simulink model "DC_Microgrid_Final"  (R2024b)
settings: Solver=VariableStepAuto  StartTime=0.0  StopTime=1.2  RelTol=1e-3
undefined symbols (not defined in the file): Ion, Lithium
libraries: spsSeriesRLCBranchLib x12, spsMeanLib x12, spsCurrentMeasurementLib x9, spsMosfetLib x9, spsIGBTDiodeLib x4, spsStairGeneratorLib x4, spsPWMGeneratorDCDCLib x4, spsVoltageMeasurementLib x3, slpidlib x3, spsDiodeLib x2, spsThreePhaseVIMeasurementLib x1, spsUniversalBridgeLib x1
settings Model: Creator=MCHJOH015  LastModifiedBy=MCHJOH015
settings SolverCC: ZeroCrossAlgorithm=Adaptive
settings DebuggingCC: MaxConsecutiveZCsMsg=none  MaskedZcDiagnostic=none  IgnoredZcDiagnostic=none

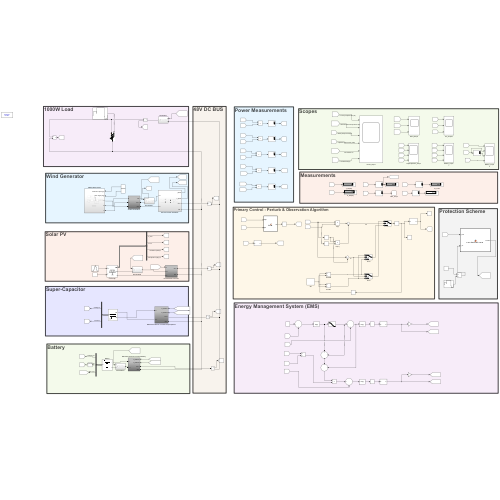
[thumbnail: Simulink's stored preview of the top-level diagram]
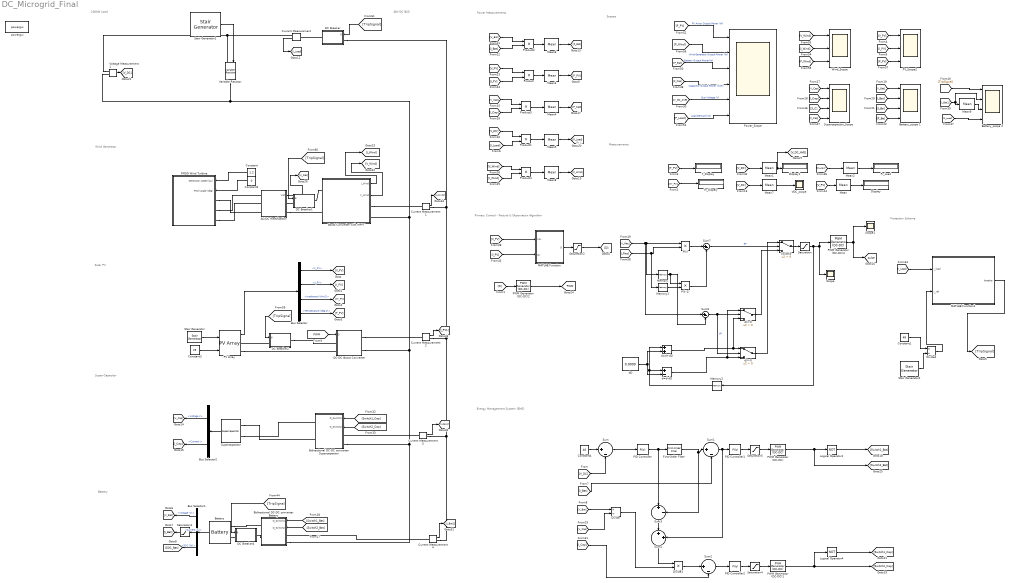
== system DC_Microgrid_Final ==
  note: Pr_L
  note: Power Measurements
  note: Scopes
  note: Protection Scheme
  note: Measurements
  note: Primary Control - Perturb & Observation Algorithm
  note: Super-Capacitor
  note: Solar PV
  note: Wind Generator
  note: 1000W Load
  note: 48V DC BUS
  note: Energy Management System (EMS)
  note: Battery
  AC/DC Rectification : Subsystem
  Battery : spsBatteryLib/Battery  BatType=Lithium-Ion  NomV=25.6  NomQ=200  SOC=50  Batt_Tr=0.1  PresetModel=on  MaxQ=200  MinV=19.2  FullV=29.7981  Dis_rate=86.9565  R=0.00128  Normal_OP=180.8696  expZone="[27.6579      9.82609]"
      settings: LibrarySourceBlock=electricdrivelib/Extra Sources/Battery
  Battery_scope 1 : Scope  NumInputPorts=4
  Battery_scope 2 : Scope  NumInputPorts=4
  Bidirectional DC-DC converter Battery : Subsystem
  Bidirectional DC-DC converter Supercapacitor : Subsystem
  Boost Converter with MPPT : Subsystem
  Bus Selector : BusSelector  OutputSignals=V_PV,I_PV,Irradiance (W/m2),Temperature (deg C)
  Bus Selector1 : BusSelector  OutputSignals=Voltage (V),Current (A),SOC (%)
  Bus Selector2 : BusSelector  OutputSignals=Voltage V,Current I
  Constant : Constant  Value=1.2
  Constant1 : Constant  Value=48
  Constant2 : Constant  Value=0
  Constant3 : Constant  Value=25
  Constant4 : Constant  Value=48
  Current Measurement{,1..4} (5 alike) : spsCurrentMeasurementLib/Current Measurement  PhasorSimulation=off  OutputType=Complex  PSBequivalent=0
  DC Breaker : Subsystem
  DC Breaker1 : Subsystem
  DC Breaker2 : Subsystem
  DC Breaker4 : Subsystem
  DC-DC Boost Converter : Subsystem
  Display : Display
  Display1 : Display
  Divide : Product  Inputs=*/
  Divide1 : Product  Inputs=**
  Divide2 : Product  Inputs=*/
  First-Order Filter : spsFirstOrderFilterLib/First-Order Filter  FilterType=Lowpass  Tc=0.015  Ts=0  Initialize=off  Vac_Init=[0, 0, 60]  Vdc_Init=0  PlotResponse=off  FreqRange="[0,  200,  1]"
  Irr_Dispaly : Display
  Logical Operator1 : Logic  Operator=NOT  IconShape=distinctive  AllPortsSameDT=off  OutDataTypeStr=boolean
  Logical Operator4 : Logic  Operator=NOT  IconShape=distinctive  AllPortsSameDT=off  OutDataTypeStr=boolean
  MATLAB Function : MATLAB Function  TreatAsAtomicUnit=on
  MATLAB Function1 : MATLAB Function  TreatAsAtomicUnit=on
  Mean{,1..9} (10 alike) : spsMeanLib/Mean  Freq=60  Vinit=0  Ts=0
  Memory : Memory  InheritSampleTime=on  LinearizeAsDelay=on
  Memory1 : Memory  InheritSampleTime=on  LinearizeAsDelay=on
  Memory2 : Memory
  P(k) : Product
  P(k-1) : Product
  PID Controller : slpidlib/PID Controller  Controller=PI  Form=Parallel  TimeDomain=Continuous-time  UseExternalTs=off  SampleTime=-1  IntegratorMethod=Forward Euler  FilterMethod=Forward Euler  ControllerParametersSource=internal  P=1.47  I=3088.21  UseKiTs=off  D=0  UseExternalDerivativeSource=off  N=100  UseFilter=on  TunerSelectOption=Transfer Function Based (PID Tuner App)  InitialConditionSource=internal  InitialConditionForIntegrator=0  InitialConditionForFilter=0  DifferentiatorICPrevScaledInput=0  ExternalReset=none  TrackingMode=off  Kt=1  LimitOutput=off  SatLimitsSource=internal  UpperSaturationLimit=inf  LowerSaturationLimit=-inf  LinearizeAsGain=on  AntiWindupMode=none  Kb=1  LimitIntegrator=off  UpperIntegratorSaturationLimit=inf  LowerIntegratorSaturationLimit=-inf  POutMin=[]  POutMax=[]  IOutMin=[]  IOutMax=[]  DOutMin=[]  DOutMax=[]  NOutMin=[]  NOutMax=[]  SumOutMin=[]  SumOutMax=[]  SaturationOutMin=[]  SaturationOutMax=[]  PParamMin=[]  PParamMax=[]  IParamMin=[]  IParamMax=[]  DParamMin=[]  DParamMax=[]  NParamMin=[]  NParamMax=[]  KbParamMin=[]  KbParamMax=[]  KtParamMin=[]  KtParamMax=[]  KbOutMin=[]  KbOutMax=[]  KtOutMin=[]  KtOutMax=[]  IntegratorOutMin=[]  IntegratorOutMax=[]  FilterOutMin=[]  FilterOutMax=[]  SumI1OutMin=[]  SumI1OutMax=[]  SumI2OutMin=[]  SumI2OutMax=[]  SumI3OutMin=[]  SumI3OutMax=[]  SumI4OutMin=[]  SumI4OutMax=[]  SumDOutMin=[]  SumDOutMax=[]  DifferentiatorOutMin=[]  DifferentiatorOutMax=[]  FilterDiffOutCoefMin=[]  FilterDiffOutCoefMax=[]  ReciprocalOutMin=[]  ReciprocalOutMax=[]  SumDenOutMin=[]  SumDenOutMax=[]  SumNumOutMin=[]  SumNumOutMax=[]  DivideOutMin=[]  DivideOutMax=[]  UdiffTsProdOutMin=[]  UdiffTsProdOutMax=[]  NTsProdOutMin=[]  NTsProdOutMax=[]  UintegralTsProdOutMin=[]  UintegralTsProdOutMax=[]  UngainTsProdOutMin=[]  UngainTsProdOutMax=[]  ClampingZeroOutDataTypeStr=Inherit: Inherit via back propagation  ClampingZeroOutMin=[]  ClampingZeroOutMax=[]  FilterDenConstantOutDataTypeStr=Inherit: Inherit via back propagation  FilterDenConstantOutMin=[]  FilterDenConstantOutMax=[]  PCopyOutDataTypeStr=Inherit: Inherit via back propagation  PCopyOutMin=[]  PCopyOutMax=[]  NCopyOutDataTypeStr=Inherit: Inherit via back propagation  NCopyOutMin=[]  NCopyOutMax=[]  IntegratorContinuousStateAttributes=''  IntegratorStateMustResolveToSignalObject=off  IntegratorRTWStateStorageClass=Auto  FilterContinuousStateAttributes=''  FilterStateMustResolveToSignalObject=off  FilterRTWStateStorageClass=Auto  ParallelPVariant=InternalParameters  IdealPVariant=Disabled  IVariant=InternalParameters  DVariant=Disabled  IntegratorVariant=Continuous  SatVariant=Disabled  AWVariant=Passthrough  PCopyVariant=Disabled  TRVariant=Disabled  FdbkBlocksVariant=Forward  IdealPFdbkVariant=Disabled  SatFdbkVariant=Disabled  DerivativeFilterVariant=Disabled  NVariant=Disabled  NCopyVariant=Disabled_SignalSpec  FilterICVariant=Disabled  IntegratorICVariant=InternalICs  ExternalResetVariant=Disabled  TRSumVariant=Passthrough  SumFdbkVariant=Disabled  SumVariant=Sum_PI  TsampFilterVariant=InternalTs  TsampNgainVariant=Passthrough  TsampIntegralVariant=Disabled_SignalSpec  ExternalSaturationOutDataTypeStr=Inherit: Same as second input  DerivativeSourceVariant=Disabled  PreIntVariant=InternalPreInt
  PID Controller1 : slpidlib/PID Controller  Controller=PI  Form=Parallel  TimeDomain=Continuous-time  UseExternalTs=off  SampleTime=-1  IntegratorMethod=Forward Euler  FilterMethod=Forward Euler  ControllerParametersSource=internal  P=0.01651  I=33.186  UseKiTs=off  D=0  UseExternalDerivativeSource=off  N=100  UseFilter=on  TunerSelectOption=Transfer Function Based (PID Tuner App)  InitialConditionSource=internal  InitialConditionForIntegrator=0  InitialConditionForFilter=0  DifferentiatorICPrevScaledInput=0  ExternalReset=none  TrackingMode=off  Kt=1  LimitOutput=off  SatLimitsSource=internal  UpperSaturationLimit=inf  LowerSaturationLimit=-inf  LinearizeAsGain=on  AntiWindupMode=none  Kb=1  LimitIntegrator=off  UpperIntegratorSaturationLimit=inf  LowerIntegratorSaturationLimit=-inf  POutMin=[]  POutMax=[]  IOutMin=[]  IOutMax=[]  DOutMin=[]  DOutMax=[]  NOutMin=[]  NOutMax=[]  SumOutMin=[]  SumOutMax=[]  SaturationOutMin=[]  SaturationOutMax=[]  PParamMin=[]  PParamMax=[]  IParamMin=[]  IParamMax=[]  DParamMin=[]  DParamMax=[]  NParamMin=[]  NParamMax=[]  KbParamMin=[]  KbParamMax=[]  KtParamMin=[]  KtParamMax=[]  KbOutMin=[]  KbOutMax=[]  KtOutMin=[]  KtOutMax=[]  IntegratorOutMin=[]  IntegratorOutMax=[]  FilterOutMin=[]  FilterOutMax=[]  SumI1OutMin=[]  SumI1OutMax=[]  SumI2OutMin=[]  SumI2OutMax=[]  SumI3OutMin=[]  SumI3OutMax=[]  SumI4OutMin=[]  SumI4OutMax=[]  SumDOutMin=[]  SumDOutMax=[]  DifferentiatorOutMin=[]  DifferentiatorOutMax=[]  FilterDiffOutCoefMin=[]  FilterDiffOutCoefMax=[]  ReciprocalOutMin=[]  ReciprocalOutMax=[]  SumDenOutMin=[]  SumDenOutMax=[]  SumNumOutMin=[]  SumNumOutMax=[]  DivideOutMin=[]  DivideOutMax=[]  UdiffTsProdOutMin=[]  UdiffTsProdOutMax=[]  NTsProdOutMin=[]  NTsProdOutMax=[]  UintegralTsProdOutMin=[]  UintegralTsProdOutMax=[]  UngainTsProdOutMin=[]  UngainTsProdOutMax=[]  ClampingZeroOutDataTypeStr=Inherit: Inherit via back propagation  ClampingZeroOutMin=[]  ClampingZeroOutMax=[]  FilterDenConstantOutDataTypeStr=Inherit: Inherit via back propagation  FilterDenConstantOutMin=[]  FilterDenConstantOutMax=[]  PCopyOutDataTypeStr=Inherit: Inherit via back propagation  PCopyOutMin=[]  PCopyOutMax=[]  NCopyOutDataTypeStr=Inherit: Inherit via back propagation  NCopyOutMin=[]  NCopyOutMax=[]  IntegratorContinuousStateAttributes=''  IntegratorStateMustResolveToSignalObject=off  IntegratorRTWStateStorageClass=Auto  FilterContinuousStateAttributes=''  FilterStateMustResolveToSignalObject=off  FilterRTWStateStorageClass=Auto  ParallelPVariant=InternalParameters  IdealPVariant=Disabled  IVariant=InternalParameters  DVariant=Disabled  IntegratorVariant=Continuous  SatVariant=Disabled  AWVariant=Passthrough  PCopyVariant=Disabled  TRVariant=Disabled  FdbkBlocksVariant=Forward  IdealPFdbkVariant=Disabled  SatFdbkVariant=Disabled  DerivativeFilterVariant=Disabled  NVariant=Disabled  NCopyVariant=Disabled_SignalSpec  FilterICVariant=Disabled  IntegratorICVariant=InternalICs  ExternalResetVariant=Disabled  TRSumVariant=Passthrough  SumFdbkVariant=Disabled  SumVariant=Sum_PI  TsampFilterVariant=InternalTs  TsampNgainVariant=Passthrough  TsampIntegralVariant=Disabled_SignalSpec  ExternalSaturationOutDataTypeStr=Inherit: Same as second input  DerivativeSourceVariant=Disabled  PreIntVariant=InternalPreInt
  PID Controller2 : slpidlib/PID Controller  Controller=PI  Form=Parallel  TimeDomain=Continuous-time  UseExternalTs=off  SampleTime=-1  IntegratorMethod=Forward Euler  FilterMethod=Forward Euler  ControllerParametersSource=internal  P=0.02303  I=77.175  UseKiTs=off  D=0  UseExternalDerivativeSource=off  N=100  UseFilter=on  TunerSelectOption=Transfer Function Based (PID Tuner App)  InitialConditionSource=internal  InitialConditionForIntegrator=0  InitialConditionForFilter=0  DifferentiatorICPrevScaledInput=0  ExternalReset=none  TrackingMode=off  Kt=1  LimitOutput=off  SatLimitsSource=internal  UpperSaturationLimit=inf  LowerSaturationLimit=-inf  LinearizeAsGain=on  AntiWindupMode=none  Kb=1  LimitIntegrator=off  UpperIntegratorSaturationLimit=inf  LowerIntegratorSaturationLimit=-inf  POutMin=[]  POutMax=[]  IOutMin=[]  IOutMax=[]  DOutMin=[]  DOutMax=[]  NOutMin=[]  NOutMax=[]  SumOutMin=[]  SumOutMax=[]  SaturationOutMin=[]  SaturationOutMax=[]  PParamMin=[]  PParamMax=[]  IParamMin=[]  IParamMax=[]  DParamMin=[]  DParamMax=[]  NParamMin=[]  NParamMax=[]  KbParamMin=[]  KbParamMax=[]  KtParamMin=[]  KtParamMax=[]  KbOutMin=[]  KbOutMax=[]  KtOutMin=[]  KtOutMax=[]  IntegratorOutMin=[]  IntegratorOutMax=[]  FilterOutMin=[]  FilterOutMax=[]  SumI1OutMin=[]  SumI1OutMax=[]  SumI2OutMin=[]  SumI2OutMax=[]  SumI3OutMin=[]  SumI3OutMax=[]  SumI4OutMin=[]  SumI4OutMax=[]  SumDOutMin=[]  SumDOutMax=[]  DifferentiatorOutMin=[]  DifferentiatorOutMax=[]  FilterDiffOutCoefMin=[]  FilterDiffOutCoefMax=[]  ReciprocalOutMin=[]  ReciprocalOutMax=[]  SumDenOutMin=[]  SumDenOutMax=[]  SumNumOutMin=[]  SumNumOutMax=[]  DivideOutMin=[]  DivideOutMax=[]  UdiffTsProdOutMin=[]  UdiffTsProdOutMax=[]  NTsProdOutMin=[]  NTsProdOutMax=[]  UintegralTsProdOutMin=[]  UintegralTsProdOutMax=[]  UngainTsProdOutMin=[]  UngainTsProdOutMax=[]  ClampingZeroOutDataTypeStr=Inherit: Inherit via back propagation  ClampingZeroOutMin=[]  ClampingZeroOutMax=[]  FilterDenConstantOutDataTypeStr=Inherit: Inherit via back propagation  FilterDenConstantOutMin=[]  FilterDenConstantOutMax=[]  PCopyOutDataTypeStr=Inherit: Inherit via back propagation  PCopyOutMin=[]  PCopyOutMax=[]  NCopyOutDataTypeStr=Inherit: Inherit via back propagation  NCopyOutMin=[]  NCopyOutMax=[]  IntegratorContinuousStateAttributes=''  IntegratorStateMustResolveToSignalObject=off  IntegratorRTWStateStorageClass=Auto  FilterContinuousStateAttributes=''  FilterStateMustResolveToSignalObject=off  FilterRTWStateStorageClass=Auto  ParallelPVariant=InternalParameters  IdealPVariant=Disabled  IVariant=InternalParameters  DVariant=Disabled  IntegratorVariant=Continuous  SatVariant=Disabled  AWVariant=Passthrough  PCopyVariant=Disabled  TRVariant=Disabled  FdbkBlocksVariant=Forward  IdealPFdbkVariant=Disabled  SatFdbkVariant=Disabled  DerivativeFilterVariant=Disabled  NVariant=Disabled  NCopyVariant=Disabled_SignalSpec  FilterICVariant=Disabled  IntegratorICVariant=InternalICs  ExternalResetVariant=Disabled  TRSumVariant=Passthrough  SumFdbkVariant=Disabled  SumVariant=Sum_PI  TsampFilterVariant=InternalTs  TsampNgainVariant=Passthrough  TsampIntegralVariant=Disabled_SignalSpec  ExternalSaturationOutDataTypeStr=Inherit: Same as second input  DerivativeSourceVariant=Disabled  PreIntVariant=InternalPreInt
  PMSG Wind Turbine : Subsystem
  PV Array : spsPVArrayLib/PV Array  Npar=8  Nser=2  PlotType=one module @ 25 deg.C & specified irradiances  S_vec="[ 1000 800 500  250 ]"  Temp_C_vec="[0 25 50  ]"  ModuleName=Waaree Energies WU-125  PlotWhenSelected=on  Pm=125.8  Ncell=72  Voc=21  Isc=8.2  Vm=17  Im=7.4  beta_Voc_pc=-0.358  alpha_Isc_pc=0.052  beta_Voc=-0.07518  alpha_Isc=0.004264  IL=8.2383  I0=2.4868e-10  nI=0.47035  Rsh=41.3301  Rs=0.19294  RobustModel=off  RobustCellTemperature=313.3991  BAL=on  Tc=Tc  Tfilter=5e-5
  PV_Scope2 : Scope  NumInputPorts=3
  PWM Generator (DC-DC) : spsPWMGeneratorDCDCLib/PWM Generator (DC-DC)  Fsw=16000  Ts=0
  PWM Generator (DC-DC)1 : spsPWMGeneratorDCDCLib/PWM Generator (DC-DC)  Fsw=16000  Ts=0
  PWM Generator (DC-DC)2 : spsPWMGeneratorDCDCLib/PWM Generator (DC-DC)  Fsw=5000  Ts=0
  PWM Generator (DC-DC)4 : spsPWMGeneratorDCDCLib/PWM Generator (DC-DC)  Fsw=5000  Ts=0
  Power_Scope : Scope  NumInputPorts=6
  Pr_Load : Display
  Product{,1..4} (5 alike) : Product
  Saturation : Saturate  UpperLimit=0.6  LowerLimit=0.2
  Saturation1 : Saturate  UpperLimit=100  LowerLimit=-100
  Saturation2 : Saturate
  Saturation4 : Saturate  UpperLimit=1  LowerLimit=0
  Saturation5 : Saturate  UpperLimit=1  LowerLimit=0
  Scope : Scope
  Scope1 : Scope
  Stair Generator : spsStairGeneratorLib/Stair Generator  t=[0.0, 0.1, 0.2, 0.3, 0.4, 0.5, 0.6, 0.7, 0.8, 0.9, 1.0, 1.1, 1.2, 1.3, 1.4, 1.5, 1.6, 1.7, 1.8, 1.9, 2.0, 2.1, 2.2, 2.3]  e=[0, 0, 0, 0, 0, 0, 0, 31, 233, 448, 631, 764, 838, 847, 790, 672, 502, 293, 78, 0, 0, 0, 0, 0]  Ts=20e-6
  Stair Generator1 : spsStairGeneratorLib/Stair Generator  t=[0.0, 0.1, 0.2, 0.3, 0.4, 0.5, 0.6, 0.7, 0.8, 0.9, 1.0, 1.1, 1.2, 1.3, 1.4, 1.5, 1.6, 1.7, 1.8, 1.9, 2.0, 2.1, 2.2, 2.3]  e=[4.13, 4.13, 5.91, 5.91, 5.91, 5.91, 5.01, 7.43, 7.43, 7.43,7.43, 7.43, 7.43, 7.43, 7.43, 7.43, 7.43, 7.43, 3.38, 2.21, 2.59, 2.59, 2.18, 4.13]  Ts=20e-6
  Stair Generator2 : spsStairGeneratorLib/Stair Generator  t=[0.0, 0.1, 0.2, 0.3, 0.4, 0.5, 0.6, 0.7, 0.8, 0.9, 1.0, 1.1, 1.2, 1.3, 1.4, 1.5, 1.6, 1.7, 1.8, 1.9, 2.0, 2.1, 2.2, 2.3]  e=[4.13, 4.13, 5.91, 5.91, 5.91, 5.91, 5.01, 7.43, 7.43, 7.43,7.43, 7.43, 7.43, 7.43, 7.43, 7.43, 7.43, 7.43, 3.38, 2.21, 2.59, 2.59, 2.18, 4.13]  Ts=20e-6
  Sum{,1..3,7..8} (6 alike) : Sum  Inputs=|+-
  Sum4 : Sum  Inputs=|++
  Supercapacitor : spsSupercapacitorLib/Supercapacitor  C=200  Rdc=.03  Voltage=32  Ns=1  Np=1  Vinit=32  Temp=25  Nc=1  r=1e-9  epsilon=6.0208e-10  Ioc=10  Vself="[48  47.8  47.06  44.65]"
      settings: LibrarySourceBlock=sps_lib/Sources/Supercapacitor
  Supercapacitor_Scope : Scope  NumInputPorts=4
  Switch3 : Switch  Criteria=u2 > Threshold  SaturateOnIntegerOverflow=off  InputSameDT=off
  T_Display : Display
  VDC_scope : Scope
  Variable Resistor : spsVariableResistorLib/Variable Resistor  Rabsmin=1e-3
      settings: LibrarySourceBlock=sps_lib/Passives/Variable Resistor
  Voltage Measurement1 : spsVoltageMeasurementLib/Voltage Measurement  PhasorSimulation=off  OutputType=Complex  PSBequivalent=0
  Wind_Scope : Scope  NumInputPorts=3
  d=d+dD : Sum
  d=d-dD : Sum  Inputs=+-
  dD : Constant  Value=0.0009
  dV<0 : Switch  Criteria=u2 > Threshold  SaturateOnIntegerOverflow=off  InputSameDT=off
  dV>0 : Switch  Criteria=u2 > Threshold  SaturateOnIntegerOverflow=off  InputSameDT=off
  powergui : sps_lib/powergui  Priority=1  SimulationMode=Discrete  SampleTime=1e-5  frequency=60  Iterations=50  frequencyindice=0  Pbase=100e6  ErrMax=1e-4  UnitsV=kV  UnitsW=MW  buscounter=0  FunctionMessages=off  echomessages=off  EnableUseOfTLC=off  CurrentSourceSwitches=off  DisableSnubberDevices=off  DisableRonSwitches=off  DisableVfSwitches=off  DisplayEquations=off  AutomaticDiscreteSolvers=off  SolverType=Tustin/Backward Euler (TBE)  Interpol=off  ExternalGateDelay=off  methode=off  Ts=100  x0status=blocks  SPID=on  SwTol=0  HookPort=off  NonlinearTolerance=1e-4  nMaxIteration=100  ContinueOnMaxIteration=off  RestoreLinks=warning  ResistiveCurrentMeasurement=off  Frange=[0:2:500]  Ylog=off  Xlog=on  ShowGrid=off  save=off  variable=ZData  structure=0  ZoomFFT=off  StartTime=0.0  cycles=1  DisplayStyle=1  fundamental=60  FreqAxis=off  MaxFrequency=1000  frequencyindicesteady=1  RmsSteady=1  display=off
  tag scope: PWM=global, pulse=global
  wires:
  [Irr_PV] -> Irr_Dispaly/1
  Bus Selector/2 -> [I_PV]  "<I_PV>"
  [V_DC] -> Mean7/1
  Bus Selector1/1 -> [V_Bat]  "<Voltage (V)>"
  Mean/1 -> Display/1
  [PWM] -> DC-DC Boost Converter/1(D)
  Voltage Measurement1/1 -> [V_DC]
  Mean2/1 -> Pr_Load/1
  [Switch2_Cap] -> Bidirectional DC-DC converter Supercapacitor/2(D_Switch2)
  [V_DC] -> Mean1/1
  Battery/1 -> Bus Selector1/1
  Bus Selector/3 -> [Irr_PV]  "<Irradiance (W/m2)>"
  [P_Load] -> Mean2/1
  [Switch2_Bat] -> Bidirectional DC-DC converter Battery/2(D_Switch2)
  Stair Generator/1 -> PV Array/1
  [T_PV] -> T_Display/1
  Bus Selector/1 -> [V_PV]  "<V_PV>"
  Mean7/1 -> VDC_scope/1
  [Switch1_Cap] -> Bidirectional DC-DC converter Supercapacitor/1(D_Switch1)
  [V_PV] -> Mean/1
  Bus Selector/4 -> [T_PV]  "<Temperature (deg C)>"
  PV Array/1 -> Bus Selector/1
  Bus Selector2/1 -> [V_Cap]  "<Voltage V>"
  Supercapacitor/1 -> Bus Selector2/1
  Mean1/1 -> [V_DC_AVE], Display1/1
  [Switch1_Bat] -> Bidirectional DC-DC converter Battery/1(D_Switch1)
  Constant2/1 -> PMSG Wind Turbine/2(Pitch angle (deg))
  Constant/1 -> PMSG Wind Turbine/1(Generator speed (pu))
  Boost Converter with MPPT/2(V_Wind) -> [V_Wind]
  Boost Converter with MPPT/1(I_Wind) -> [I_Wind]
  Product2/1 -> Mean6/1
  Product/1 -> Mean3/1
  Product3/1 -> Mean4/1
  Product4/1 -> Mean8/1
  Product1/1 -> Mean5/1
  [I_Cap] -> Supercapacitor_Scope/2
  [V_Wind] -> Wind_Scope/1
  [I_Bat] -> Battery_scope 1/2
  [S_C] -> Supercapacitor_Scope/3
  [P_Ba] -> Battery_scope 1/4
  [P_Wind] -> Wind_Scope/3
  [P_PV] -> PV_Scope2/3
  [V_PV] -> PV_Scope2/1
  [V_Cap] -> Supercapacitor_Scope/1
  [I_PV] -> PV_Scope2/2
  [S_Ba] -> Battery_scope 1/3
  [I_Wind] -> Wind_Scope/2
  [P_Cap] -> Supercapacitor_Scope/4
  [V_Bat] -> Battery_scope 1/1
  Saturation2/1 -> [D]
  [D] -> PWM Generator (DC-DC)2/1
  MATLAB Function/1(D) -> Saturation2/1
  [V_Bat] -> Product2/1
  [V_PV] -> Product/1
  [I_PV] -> Product/2
  [V_Cap] -> Product3/1
  [I_Cap] -> Product3/2
  [V_DC] -> Product1/1
  [I_Load] -> Product1/2
  [I_Wind] -> Product4/2
  [V_Wind] -> Product4/1
  Mean6/1 -> [P_Bat]
  Mean3/1 -> [P_PV]
  Mean4/1 -> [P_Cap]
  Mean5/1 -> [P_Load]
  Mean8/1 -> [P_Wind]
  [I_PV] -> MATLAB Function/2(Ipv)
  [V_PV] -> MATLAB Function/1(Vpv)
  Bus Selector1/3 -> [SOC_Bat]  "<SOC (%)>"
  [I_Bat] -> Product2/2
  Bus Selector2/2 -> [I_Cap]  "<Current I>"
  Memory/1 -> Sum8/2, P(k-1)/1
  d=d+dD/1 -> dV<0/3, dV>0/1
  [I_Rec] -> Memory1/1, P(k)/2
  dV<0/1 -> Switch3/3
  d=d-dD/1 -> dV<0/1, dV>0/3
  Sum7/1 -> Switch3/2  "dP"
  P(k)/1 -> Sum7/1
  Memory2/1 -> d=d-dD/1, d=d+dD/1
  Switch3/1 -> Saturation/1
  P(k-1)/1 -> Sum7/2
  Memory1/1 -> P(k-1)/2
  Sum8/1 -> dV>0/2, dV<0/2  "dV"
  dD/1 -> d=d-dD/2, d=d+dD/2
  [V_Rec] -> Sum8/1, Memory/1, P(k)/1
  dV>0/1 -> Switch3/1
  Saturation/1 -> PWM Generator (DC-DC)4/1, Scope/1, Memory2/1
  PWM Generator (DC-DC)4/1 -> Scope1/1, [pulse]
  AC/DC Rectification/1(Vdc) -> [V_Rec]
  Constant3/1 -> PV Array/2
  Current Measurement/1 -> [I_Load]
  Stair Generator1/1 -> Variable Resistor/1
  Saturation1/1 -> [I_Bat]
  Bus Selector1/2 -> Saturation1/1  "<Current (A)>"
  [P_PV] -> Power_Scope/1  "PV Array Output Power (W)"
  [P_Wind] -> Power_Scope/2  "Wind Generator Output Power (W)"
  [P_Bat] -> Power_Scope/3  "Battery Output Power(W)"
  [P_Cap] -> Power_Scope/4  "Capacitor Output Power (VAR)"
  [V_DC_AVE] -> Power_Scope/5  "Bus Voltage (V)"
  [P_Load] -> Power_Scope/6  "Load Demand (W)"
  [I_Bat] -> Sum1/2
  Sum2/1 -> PID Controller2/1
  Sum1/1 -> PID Controller1/1, Sum4/2
  Constant4/1 -> Sum/1
  Logical Operator4/1 -> [Switch1_Cap]
  Sum/1 -> PID Controller/1
  Divide/1 -> Divide1/2
  PID Controller1/1 -> Saturation5/1
  Divide1/1 -> Sum2/1
  [V_DC] -> Sum/2
  PID Controller/1 -> First-Order Filter/1, Sum3/1
  Logical Operator1/1 -> [Switch1_Bat]
  Sum4/1 -> Divide1/1
  [I_Cap] -> Sum2/2
  Saturation5/1 -> PWM Generator (DC-DC)/1
  PID Controller2/1 -> Saturation4/1
  [V_Bat] -> Divide/1
  PWM Generator (DC-DC)/1 -> [Switch2_Bat], Logical Operator1/1
  [V_Cap] -> Divide/2
  Sum3/1 -> Sum4/1
  PWM Generator (DC-DC)1/1 -> [Switch2_Cap], Logical Operator4/1
  Saturation4/1 -> PWM Generator (DC-DC)1/1
  First-Order Filter/1 -> Sum3/2, Sum1/1
  Current Measurement4/1 -> [I_Bat1]
  Current Measurement3/1 -> [I_Cap1]
  Current Measurement2/1 -> [I_PV1]
  Current Measurement1/1 -> [I_Wind1]
  PWM Generator (DC-DC)2/1 -> [PWM]
  MATLAB Function1/1(breaker) -> [TripSignal]
  [TripSignal] -> DC Breaker4/1(g)
  [TripSignal] -> DC Breaker2/1(g)
  [TripSignal] -> DC Breaker1/1(g)
  [TripSignal] -> DC Breaker/1(g)
  [I_Load] -> MATLAB Function1/1(I_load)
  Divide2/1 -> MATLAB Function1/2(I_ref)
  Constant1/1 -> Divide2/1
  Stair Generator2/1 -> Divide2/2
  [TripSignal] -> Battery_scope 2/1
  [I_Bat1] -> Battery_scope 2/2, Mean9/1
  [P_Load] -> Battery_scope 2/4
  Mean9/1 -> Battery_scope 2/3
  connections:
  Bidirectional DC-DC converter Battery/LConn2 -- Bidirectional DC-DC converter Supercapacitor/LConn2 -- DC-DC Boost Converter/RConn2 -- Variable Resistor/RConn1 -- Voltage Measurement1/LConn2 -- Boost Converter with MPPT/RConn2
  Voltage Measurement1/LConn1 -- Variable Resistor/LConn1 -- Current Measurement/RConn1
  PV Array/RConn2 -- DC-DC Boost Converter/LConn2
  Battery/LConn2 -- Bidirectional DC-DC converter Battery/RConn1
  Current Measurement4/RConn1 -- Current Measurement3/RConn1 -- DC Breaker/LConn1 -- Current Measurement1/RConn1 -- Current Measurement2/RConn1
  PMSG Wind Turbine/LConn2 -- AC/DC Rectification/LConn1
  PMSG Wind Turbine/LConn1 -- AC/DC Rectification/LConn3
  PMSG Wind Turbine/LConn3 -- AC/DC Rectification/LConn2
  AC/DC Rectification/RConn2 -- Boost Converter with MPPT/LConn2
  Supercapacitor/LConn2 -- Bidirectional DC-DC converter Supercapacitor/RConn1
  Boost Converter with MPPT/RConn1 -- Current Measurement1/LConn1
  DC-DC Boost Converter/RConn1 -- Current Measurement2/LConn1
  Current Measurement3/LConn1 -- Bidirectional DC-DC converter Supercapacitor/LConn1
  Current Measurement4/LConn1 -- Bidirectional DC-DC converter Battery/LConn1
  DC Breaker/RConn1 -- Current Measurement/LConn1
  DC Breaker1/LConn1 -- AC/DC Rectification/RConn1
  Boost Converter with MPPT/LConn1 -- DC Breaker1/RConn1
  DC Breaker2/LConn1 -- PV Array/RConn1
  DC Breaker2/RConn1 -- DC-DC Boost Converter/LConn1
  DC Breaker4/LConn1 -- Battery/LConn1
  DC Breaker4/RConn1 -- Bidirectional DC-DC converter Battery/RConn2
  Supercapacitor/LConn1 -- Bidirectional DC-DC converter Supercapacitor/RConn2

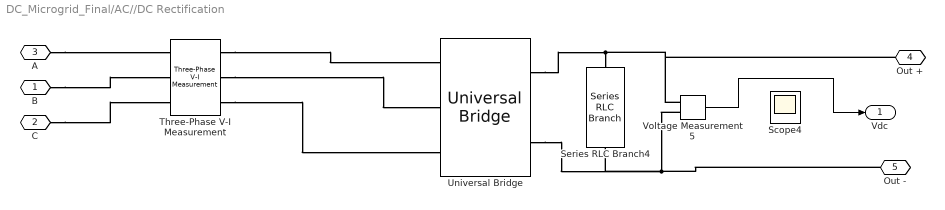
== system DC_Microgrid_Final/AC//DC Rectification ==
  Scope4 : Scope
  Series RLC Branch4 : spsSeriesRLCBranchLib/Series RLC Branch  LConnTagsString=__new0  RConnTagsString=__new0  BranchType=C  Resistance=1  Inductance=1e-3  SetiL0=off  InitialCurrent=0  Capacitance=11000e-6  Setx0=off  InitialVoltage=0  Measurements=None
  Three-Phase V-I Measurement : spsThreePhaseVIMeasurementLib/Three-Phase V-I Measurement  VoltageMeasurement=no  SetLabelV=off  LabelV=Vabc  Vpu=off  VpuLL=off  CurrentMeasurement=no  SetLabelI=off  LabelI=Iabc  Ipu=off  Pbase=100e6  Vbase=500e3  OutputType=Complex  PhasorSimulation=off  PSBequivalent=0
  Universal Bridge : spsUniversalBridgeLib/Universal Bridge  Arms=3  SnubberResistance=1e5  SnubberCapacitance=inf  Device=Diodes  Ron=1e-3  Lon=0  ForwardVoltages="[  0  0  ]"  ForwardVoltage=0  GTOparameters=[ 10e-6 , 20e-6 ]  IGBTparameters=[ 1e-6 , 2e-6 ]  Measurements=None  Measurements_2=None  converterType=Rectifier
  Voltage Measurement5 : spsVoltageMeasurementLib/Voltage Measurement  PhasorSimulation=off  OutputType=Complex  PSBequivalent=0
  B : PMIOPort  Side=Left
  C : PMIOPort  Port=2  Side=Left
  A : PMIOPort  Port=3  Side=Left
  Out + : PMIOPort  Port=4  Side=Right
  Out - : PMIOPort  Port=5  Side=Right
  Vdc : Outport
  wires:
  Voltage Measurement5/1 -> Vdc/1
  connections:
  Voltage Measurement5/LConn2 -- Out -/RConn1 -- Universal Bridge/RConn2 -- Series RLC Branch4/RConn1
  Universal Bridge/RConn1 -- Out +/RConn1 -- Voltage Measurement5/LConn1 -- Series RLC Branch4/LConn1
  Three-Phase V-I Measurement/RConn3 -- Universal Bridge/LConn3
  Three-Phase V-I Measurement/RConn1 -- Universal Bridge/LConn1
  Three-Phase V-I Measurement/RConn2 -- Universal Bridge/LConn2
  A/RConn1 -- Three-Phase V-I Measurement/LConn1
  B/RConn1 -- Three-Phase V-I Measurement/LConn2
  C/RConn1 -- Three-Phase V-I Measurement/LConn3

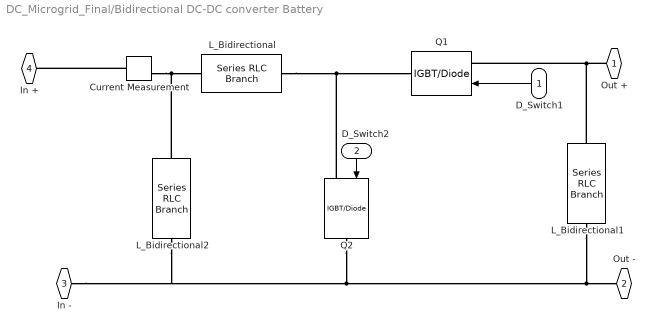
== system DC_Microgrid_Final/Bidirectional DC-DC converter Battery ==
  D_Switch1 : Inport
  D_Switch2 : Inport  Port=2
  Current Measurement : spsCurrentMeasurementLib/Current Measurement  PhasorSimulation=off  OutputType=Complex  PSBequivalent=0
  L_Bidirectional : spsSeriesRLCBranchLib/Series RLC Branch  LConnTagsString=__new0  RConnTagsString=__new0  BranchType=RL  Resistance=0.05  Inductance=82e-6  SetiL0=off  InitialCurrent=0  Capacitance=1e-6  Setx0=off  InitialVoltage=0  Measurements=None
  L_Bidirectional1 : spsSeriesRLCBranchLib/Series RLC Branch  LConnTagsString=__new0  RConnTagsString=__new0  BranchType=C  Resistance=0.05  Inductance=0.3e-3  SetiL0=off  InitialCurrent=0  Capacitance=1800e-6  Setx0=off  InitialVoltage=0  Measurements=None
  L_Bidirectional2 : spsSeriesRLCBranchLib/Series RLC Branch  LConnTagsString=__new0  RConnTagsString=__new0  BranchType=RC  Resistance=0.05  Inductance=0.3e-3  SetiL0=off  InitialCurrent=0  Capacitance=150e-6  Setx0=off  InitialVoltage=0  Measurements=None
  Q1 : spsIGBTDiodeLib/IGBT//Diode  Ron=1e-3  Rs=1e5  Cs=inf  Measurements=off
  Q2 : spsIGBTDiodeLib/IGBT//Diode  Ron=1e-3  Rs=1e5  Cs=inf  Measurements=off
  Out + : PMIOPort  Side=Left
  Out - : PMIOPort  Port=2  Side=Left
  In - : PMIOPort  Port=3  Side=Right
  In + : PMIOPort  Port=4  Side=Right
  wires:
  D_Switch2/1 -> Q2/1
  D_Switch1/1 -> Q1/1
  connections:
  Q2/RConn1 -- In -/RConn1 -- L_Bidirectional2/LConn1 -- L_Bidirectional1/LConn1 -- Out -/RConn1
  Out +/RConn1 -- Q1/LConn1 -- L_Bidirectional1/RConn1
  Q2/LConn1 -- L_Bidirectional/LConn1 -- Q1/RConn1
  Current Measurement/LConn1 -- In +/RConn1
  Current Measurement/RConn1 -- L_Bidirectional/RConn1 -- L_Bidirectional2/RConn1

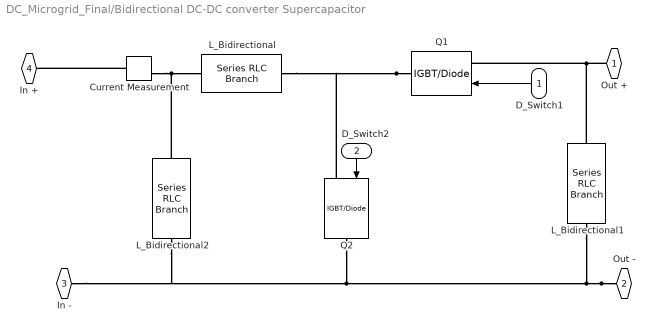
== system DC_Microgrid_Final/Bidirectional DC-DC converter Supercapacitor ==
  D_Switch1 : Inport
  D_Switch2 : Inport  Port=2
  Current Measurement : spsCurrentMeasurementLib/Current Measurement  PhasorSimulation=off  OutputType=Complex  PSBequivalent=0
  L_Bidirectional : spsSeriesRLCBranchLib/Series RLC Branch  LConnTagsString=__new0  RConnTagsString=__new0  BranchType=RL  Resistance=0.05  Inductance=68e-6  SetiL0=off  InitialCurrent=0  Capacitance=1e-6  Setx0=off  InitialVoltage=0  Measurements=None
  L_Bidirectional1 : spsSeriesRLCBranchLib/Series RLC Branch  LConnTagsString=__new0  RConnTagsString=__new0  BranchType=C  Resistance=0.05  Inductance=0.3e-3  SetiL0=off  InitialCurrent=0  Capacitance=2200e-6  Setx0=off  InitialVoltage=0  Measurements=None
  L_Bidirectional2 : spsSeriesRLCBranchLib/Series RLC Branch  LConnTagsString=__new0  RConnTagsString=__new0  BranchType=C  Resistance=0.05  Inductance=0.3e-3  SetiL0=off  InitialCurrent=0  Capacitance=220e-6  Setx0=off  InitialVoltage=0  Measurements=None
  Q1 : spsIGBTDiodeLib/IGBT//Diode  Ron=1e-3  Rs=1e5  Cs=inf  Measurements=off
  Q2 : spsIGBTDiodeLib/IGBT//Diode  Ron=1e-3  Rs=1e5  Cs=inf  Measurements=off
  Out + : PMIOPort  Side=Left
  Out - : PMIOPort  Port=2  Side=Left
  In - : PMIOPort  Port=3  Side=Right
  In + : PMIOPort  Port=4  Side=Right
  wires:
  D_Switch2/1 -> Q2/1
  D_Switch1/1 -> Q1/1
  connections:
  Out -/RConn1 -- In -/RConn1 -- L_Bidirectional2/LConn1 -- Q2/RConn1 -- L_Bidirectional1/LConn1
  Current Measurement/RConn1 -- L_Bidirectional/RConn1 -- L_Bidirectional2/RConn1
  Out +/RConn1 -- Q1/LConn1 -- L_Bidirectional1/RConn1
  Q1/RConn1 -- Q2/LConn1 -- L_Bidirectional/LConn1
  Current Measurement/LConn1 -- In +/RConn1

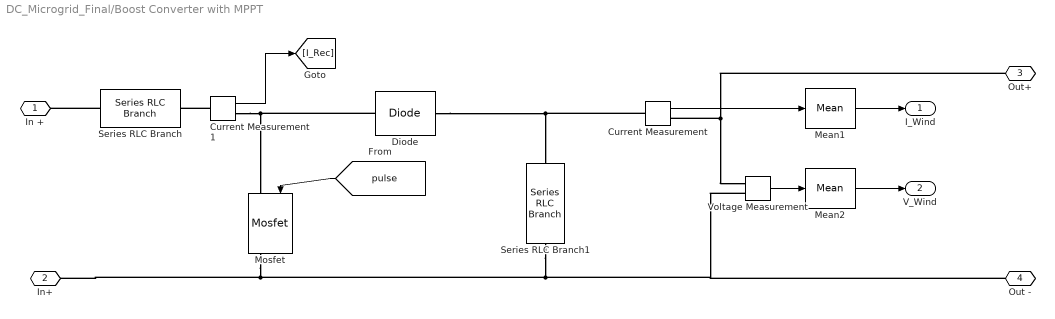
== system DC_Microgrid_Final/Boost Converter with MPPT ==
  Current Measurement : spsCurrentMeasurementLib/Current Measurement  PhasorSimulation=off  OutputType=Complex  PSBequivalent=0
  Current Measurement1 : spsCurrentMeasurementLib/Current Measurement  PhasorSimulation=off  OutputType=Complex  PSBequivalent=0
  Diode : spsDiodeLib/Diode  Ron=0.001  Lon=0  Vf=0.8  IC=0  UseSnubber=0  Rs=500  Cs=250e-9  Measurements=off
  Mean1 : spsMeanLib/Mean  Freq=50  Vinit=0  Ts=50e-6
  Mean2 : spsMeanLib/Mean  Freq=50  Vinit=0  Ts=50e-6
  Mosfet : spsMosfetLib/Mosfet  Ron=0.1  Lon=0  Rd=0.01  Vfd=0  IC=0  Rs=1e5  Cs=inf  Measurements=on
  Series RLC Branch : spsSeriesRLCBranchLib/Series RLC Branch  LConnTagsString=__new0  RConnTagsString=__new0  BranchType=RL  Resistance=1  Inductance=20e-6  SetiL0=off  InitialCurrent=0  Capacitance=1e-6  Setx0=off  InitialVoltage=0  Measurements=None
  Series RLC Branch1 : spsSeriesRLCBranchLib/Series RLC Branch  LConnTagsString=__new0  RConnTagsString=__new0  BranchType=C  Resistance=1  Inductance=1e-3  SetiL0=off  InitialCurrent=0  Capacitance=1500e-6  Setx0=off  InitialVoltage=0  Measurements=None
  Voltage Measurement : spsVoltageMeasurementLib/Voltage Measurement  PhasorSimulation=off  OutputType=Complex  PSBequivalent=0
  In + : PMIOPort  Side=Left
  In+ : PMIOPort  Port=2  Side=Left
  "Out+ " : PMIOPort  Port=3  Side=Right
  Out - : PMIOPort  Port=4  Side=Right
  I_Wind : Outport
  V_Wind : Outport  Port=2
  wires:
  [pulse] -> Mosfet/1
  Mean1/1 -> I_Wind/1
  Voltage Measurement/1 -> Mean2/1
  Mean2/1 -> V_Wind/1
  Current Measurement/1 -> Mean1/1
  Current Measurement1/1 -> [I_Rec]
  connections:
  Diode/RConn1 -- Current Measurement/LConn1 -- Series RLC Branch1/LConn1
  Diode/LConn1 -- Current Measurement1/RConn1 -- Mosfet/LConn1
  Current Measurement1/LConn1 -- Series RLC Branch/RConn1
  Series RLC Branch1/RConn1 -- Out -/RConn1 -- Voltage Measurement/LConn2 -- Mosfet/RConn1 -- In+/RConn1
  Series RLC Branch/LConn1 -- In +/RConn1
  "Out+ "/RConn1 -- Voltage Measurement/LConn1 -- Current Measurement/RConn1

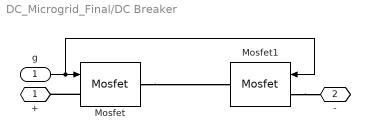
== system DC_Microgrid_Final/DC Breaker ==
  g : Inport
  Mosfet : spsMosfetLib/Mosfet  Ron=0.1  Lon=0  Rd=0.01  Vfd=0  IC=0  Rs=1e5  Cs=inf  Measurements=off
  Mosfet1 : spsMosfetLib/Mosfet  Ron=0.1  Lon=0  Rd=0.01  Vfd=0  IC=0  Rs=1e5  Cs=inf  Measurements=off
  + : PMIOPort  Side=Left
  - : PMIOPort  Port=2  Side=Right
  wires:
  g/1 -> Mosfet1/1, Mosfet/1
  connections:
  Mosfet/RConn1 -- Mosfet1/RConn1
  Mosfet1/LConn1 -- -/RConn1
  Mosfet/LConn1 -- +/RConn1

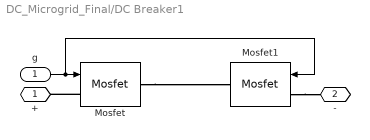
== system DC_Microgrid_Final/DC Breaker1 ==
  g : Inport
  Mosfet : spsMosfetLib/Mosfet  Ron=0.1  Lon=0  Rd=0.01  Vfd=0  IC=0  Rs=1e5  Cs=inf  Measurements=off
  Mosfet1 : spsMosfetLib/Mosfet  Ron=0.1  Lon=0  Rd=0.01  Vfd=0  IC=0  Rs=1e5  Cs=inf  Measurements=off
  + : PMIOPort  Side=Left
  - : PMIOPort  Port=2  Side=Right
  wires:
  g/1 -> Mosfet1/1, Mosfet/1
  connections:
  Mosfet/RConn1 -- Mosfet1/RConn1
  Mosfet1/LConn1 -- -/RConn1
  Mosfet/LConn1 -- +/RConn1

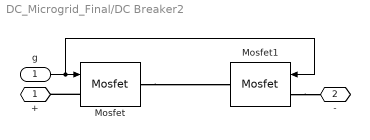
== system DC_Microgrid_Final/DC Breaker2 ==
  g : Inport
  Mosfet : spsMosfetLib/Mosfet  Ron=0.1  Lon=0  Rd=0.01  Vfd=0  IC=0  Rs=1e5  Cs=inf  Measurements=off
  Mosfet1 : spsMosfetLib/Mosfet  Ron=0.1  Lon=0  Rd=0.01  Vfd=0  IC=0  Rs=1e5  Cs=inf  Measurements=off
  + : PMIOPort  Side=Left
  - : PMIOPort  Port=2  Side=Right
  wires:
  g/1 -> Mosfet1/1, Mosfet/1
  connections:
  Mosfet/RConn1 -- Mosfet1/RConn1
  Mosfet1/LConn1 -- -/RConn1
  Mosfet/LConn1 -- +/RConn1

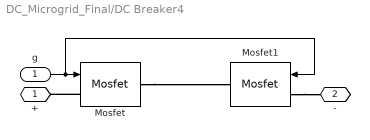
== system DC_Microgrid_Final/DC Breaker4 ==
  g : Inport
  Mosfet : spsMosfetLib/Mosfet  Ron=0.1  Lon=0  Rd=0.01  Vfd=0  IC=0  Rs=1e5  Cs=inf  Measurements=off
  Mosfet1 : spsMosfetLib/Mosfet  Ron=0.1  Lon=0  Rd=0.01  Vfd=0  IC=0  Rs=1e5  Cs=inf  Measurements=off
  + : PMIOPort  Side=Left
  - : PMIOPort  Port=2  Side=Right
  wires:
  g/1 -> Mosfet1/1, Mosfet/1
  connections:
  Mosfet/RConn1 -- Mosfet1/RConn1
  Mosfet1/LConn1 -- -/RConn1
  Mosfet/LConn1 -- +/RConn1

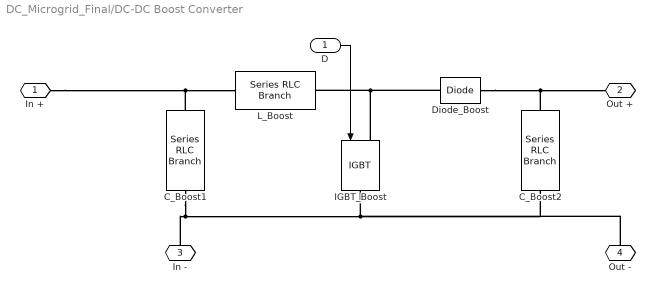
== system DC_Microgrid_Final/DC-DC Boost Converter ==
  D : Inport
  C_Boost1 : spsSeriesRLCBranchLib/Series RLC Branch  LConnTagsString=__new0  RConnTagsString=__new0  BranchType=C  Resistance=0.01  Inductance=1e-3  SetiL0=off  InitialCurrent=0  Capacitance=1000e-6  Setx0=off  InitialVoltage=0  Measurements=None
  C_Boost2 : spsSeriesRLCBranchLib/Series RLC Branch  LConnTagsString=__new0  RConnTagsString=__new0  BranchType=C  Resistance=0.01  Inductance=1e-3  SetiL0=off  InitialCurrent=0  Capacitance=1100e-6  Setx0=off  InitialVoltage=0  Measurements=None
  Diode_Boost : spsDiodeLib/Diode  Ron=1e-4  Lon=0  Vf=0  IC=0  UseSnubber=off  Rs=inf  Cs=inf  Measurements=off
  IGBT_Boost : spsIGBTLib/IGBT  Ron=0.001  Lon=0  Vf=0  Tf=0  Tt=0  IC=0  Rs=1e5  Cs=inf  Measurements=off
  L_Boost : spsSeriesRLCBranchLib/Series RLC Branch  LConnTagsString=__new0  RConnTagsString=__new0  BranchType=RL  Resistance=0.05  Inductance=100e-6  SetiL0=off  InitialCurrent=0  Capacitance=1e-6  Setx0=off  InitialVoltage=0  Measurements=None
  In + : PMIOPort  Side=Left
  Out + : PMIOPort  Port=2  Side=Right
  In - : PMIOPort  Port=3  Side=Left
  Out - : PMIOPort  Port=4  Side=Right
  wires:
  D/1 -> IGBT_Boost/1
  connections:
  IGBT_Boost/LConn1 -- Diode_Boost/LConn1 -- L_Boost/RConn1
  Diode_Boost/RConn1 -- C_Boost2/LConn1 -- Out +/RConn1
  In +/RConn1 -- C_Boost1/LConn1 -- L_Boost/LConn1
  In -/RConn1 -- C_Boost1/RConn1 -- C_Boost2/RConn1 -- Out -/RConn1 -- IGBT_Boost/RConn1

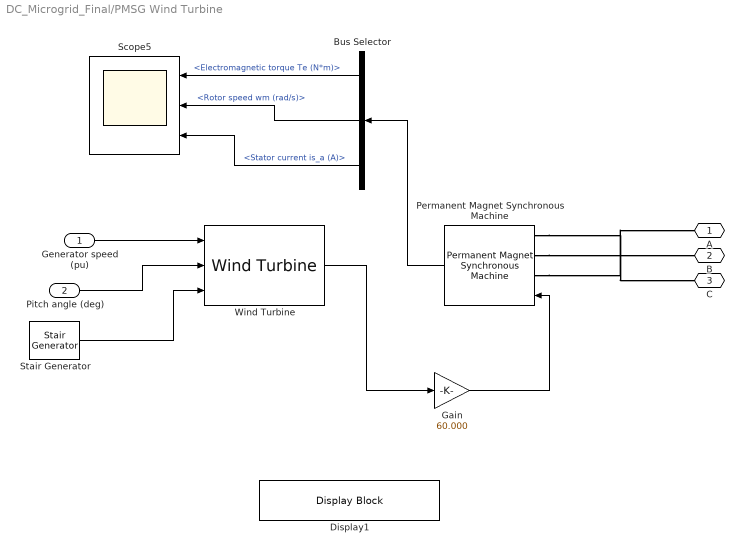
== system DC_Microgrid_Final/PMSG Wind Turbine ==
  Generator speed (pu) : Inport
  Pitch angle (deg) : Inport  Port=2
  Bus Selector : BusSelector  OutputSignals=Electromagnetic torque Te (N*m),Rotor speed wm (rad/s),Stator current is_a (A)
  Display1 : DisplayBlock  LabelPosition=Hide  Transparency=1
  Gain : Gain  Gain=60.000
  Permanent Magnet Synchronous Machine : spsPermanentMagnetSynchronousMachineLib/Permanent Magnet Synchronous Machine  NbPhases=3  FluxDistribution=Sinusoidal  RotorType=Salient-pole  MechanicalLoad=Torque Tm  PresetModel="14:  67.27 Nm 560 Vdc 1700 RPM - 70.2 Nm"  ShowDetailedParameters=on  MeasurementBus=off  Resistance=0.085  Inductance=8.5e-3  dqInductances=[0.0009025 0.0009975]  La=0.000395  MachineConstant=Flux linkage established by magnets (V.s)  Flux=0.192  VoltageCst=139.2998  TorqueCst=1.152  Flat=120  Mechanical=[0.008 0.001147 4 0]  PolePairs=4  InitialConditions=[0,0, 0,0]  InitialConditions5ph=[0 0 0 0 0 0]  RefAngle=90 degrees behind phase A axis (modified Park)  IterativeDiscreteModel=Trapezoidal non iterative  TsBlock=-1  TsPowergui=0
  Scope5 : Scope  NumInputPorts=3
  Stair Generator : spsStairGeneratorLib/Stair Generator  t=[0.0, 0.1, 0.2, 0.3, 0.4, 0.5, 0.6, 0.7, 0.8, 0.9, 1.0, 1.1, 1.2, 1.3, 1.4, 1.5, 1.6, 1.7, 1.8, 1.9, 2.0, 2.1, 2.2, 2.3]  e=[4.3, 4.2, 3.9, 5.7, 7.5, 8.6, 9.7, 9.5, 8.2, 7.0, 5.7, 5.2, 4.7, 4.8, 5.6, 6.5, 7.2, 8.0, 8.9, 9.2, 8.5, 7.6, 6.7, 6.0]  Ts=20e-6
  Wind Turbine : spsWindTurbineLib/Wind Turbine  Pnom=1e3  Pelec_base=1e3/0.9  wind_base=8  P_wind_base=0.85  speed_nom=1.2  pitch_angle=0  c1_c6="[0.51763          116          0.4            5           21     0.006795]"  cp_nom=0.48  lambda_nom=8.1
  A : PMIOPort  Side=Left
  B : PMIOPort  Port=2  Side=Left
  C : PMIOPort  Port=3  Side=Left
  wires:
  Permanent Magnet Synchronous Machine/1 -> Bus Selector/1
  Bus Selector/2 -> Scope5/2  "<Rotor speed wm (rad/s)>"
  Bus Selector/1 -> Scope5/1  "<Electromagnetic torque Te (N*m)>"
  Generator speed (pu)/1 -> Wind Turbine/1
  Bus Selector/3 -> Scope5/3  "<Stator current is_a (A)>"
  Wind Turbine/1 -> Gain/1
  Gain/1 -> Permanent Magnet Synchronous Machine/1
  Stair Generator/1 -> Wind Turbine/3
  Pitch angle (deg)/1 -> Wind Turbine/2
  connections:
  Permanent Magnet Synchronous Machine/LConn3 -- C/RConn1
  Permanent Magnet Synchronous Machine/LConn1 -- A/RConn1
  Permanent Magnet Synchronous Machine/LConn2 -- B/RConn1

== matlab function DC_Microgrid_Final/MATLAB Function ==
  settings: updateMethod=DISCRETE  sampleTime=1e-4
  data: Vpv input; D output; Ipv input
function D = PandO(Vpv,Ipv)

persistent Dold Pold Vold


if isempty(Dold)
    Dold = 0.35;
    Vold = 17;
    Pold = 120;
end


deltaD = 0.001;

Ppv = Vpv*Ipv;

if (Ppv-Pold) ~= 0
    if (Ppv-Pold) > 0
        if (Vpv-Vold) > 0
            D = Dold - deltaD;
        else
            D = Dold + deltaD;
        end
    else
        if (Vpv-Vold) > 0
            D = Dold + deltaD;
        else
            D = Dold - deltaD;
        end        
    end
else
    D = Dold;
end

Dold = D;
Vold = Vpv;
Pold = Ppv;

== matlab function DC_Microgrid_Final/MATLAB Function1 ==
  data: I_load input; breaker output; I_ref input
function breaker = CurrentDerivativeProtection(I_load, I_ref)
% Fast di/dt + overcurrent protection with debounce.
% No auto-reclose: once tripped, breaker stays open until reset externally.
%
% breaker = 1 (closed/on), 0 (tripped/off)

%% Simulation Time Scaling
S  = 36000;     % real_time = S * sim_time
Ts = 1e-4;      % Simulink sample time

%% Protection Settings (Real-World Time Base)
tau_real         = 1e-3;    % Current filter time constant (1 ms)
t_db_real        = 0.5e-3;  % Debounce before tripping (0.5 ms)
theta_trip_real  = 5e6;     % di/dt trip level [A/s]
OC_trip_mult     = 1.50;    % Trip if |I| > 150% of expected current

%% Convert to Sim-Time
Ts_real = Ts * S;
alpha   = Ts_real / (tau_real + Ts_real); % Filter coefficient

%% Internal States
persistent i_f_prev breaker_state db_real
if isempty(i_f_prev)
    i_f_prev      = 0;
    breaker_state = 1;   % Start closed
    db_real       = 0;
end

%% 1) Filter Current
i_f = i_f_prev + alpha * (I_load - i_f_prev);

%% 2) di/dt in Real Units
di_dt_real = (i_f - i_f_prev) / Ts_real;

%% 3) Trip Decision with Debounce
% Check di/dt threshold
trip_request = (abs(di_dt_real) >= theta_trip_real);

% Overcurrent check based on rated reference
I_trip_real = OC_trip_mult * I_ref;
trip_request = trip_request || (abs(i_f) >= I_trip_real);

% Only trip if breaker is still closed
if breaker_state == 1
    if trip_request
        db_real = db_real + Ts_real;
        if db_real >= t_db_real
            breaker_state = 0;   % Trip
            db_real       = 0;
        end
    else
        db_real = 0;             % Reset debounce if condition clears
    end
end

%% Output
breaker  = breaker_state;
i_f_prev = i_f;

end
